simulink model "Accelerator"  (R2022b)
settings: Solver=FixedStepDiscrete  StartTime=0.0  StopTime=10  FixedStep=0.005  RelTol=1e-3  EnableMultiTasking=on
PreLoadFcn:
  | try, model_open; catch, disp('Error occurred while executing model pre-load callback: model_open.m'); disp('Please assure that the MATLAB working directory is set to the model directory before opening.'); end
InitFcn:
  | try, model_open; catch, end
undefined symbols (not defined in the file): GCM, raptor_get_safe_string, raptor_xcp_function
libraries: Raptor_lib x134, simulink x14, Blocks_Library x2, simulink_extras x1
(part 3 of 3)

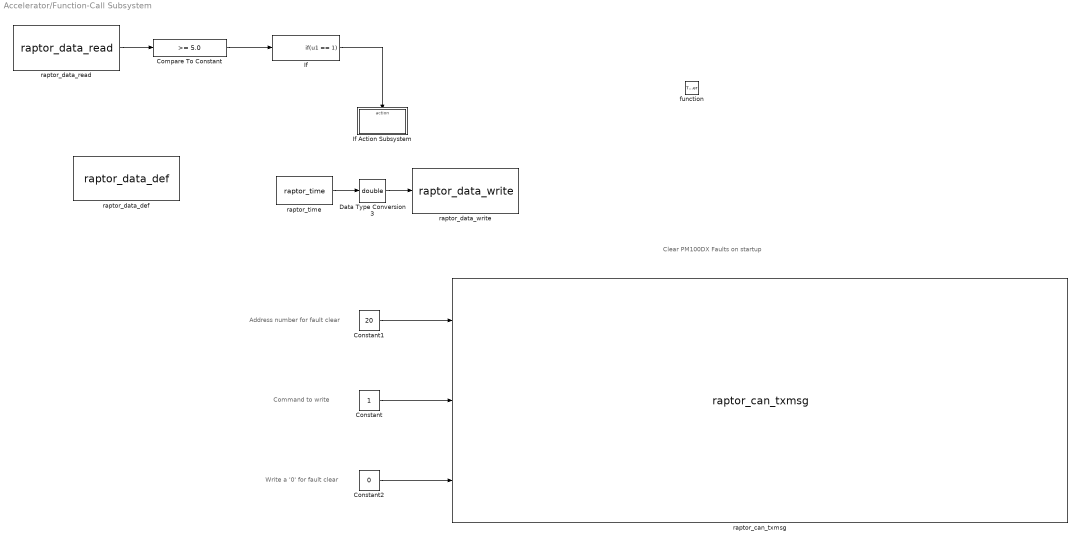
== system Accelerator/Function-Call Subsystem ==
  note: Write a '0' for fault clear
  note: Command to write
  note: Address number for fault clear
  note: Clear PM100DX Faults on startup
  function : TriggerPort  TriggerType=function-call  VariantControl=(inherit)
  Compare To Constant : simulink/Logic and Bit Operations/Compare To Constant  relop=>=  const=5.0  OutDataTypeStr=boolean
  Constant : Constant
  Constant1 : Constant  Value=20
  Constant2 : Constant  Value=0
  Data Type Conversion3 : DataTypeConversion  OutDataTypeStr=double  SaturateOnIntegerOverflow=off  RndMeth=Floor
  If : If  IfExpression=u1 == 1  ShowElse=off
  If Action Subsystem : Subsystem  TreatAsAtomicUnit=on
  raptor_can_txmsg : Raptor_lib/CAN/raptor_can_txmsg  canDefinition=struct('dbcFile', '20210505 RMS PM and RM CAN DB.dbc','message', 'M193_Read_Write_Param_Command','comment', 'Parameter Message sent as needed by VCU to request info, change EEPROM, or command a function.','signals', {{'D1_Parameter_Address_Command','D2_Read_Write_Command','D3_Data_Command'}},'enabled', [ 1 1 1;],'scaled', [ 1 1 1;],'canBus', '''CAN1''','messageID', [ 193;],'idMask', [ 536870911;],'payloadMask', [],'payloadValue', [],'period', [ 0;],'queueSize', [ 1;],'label', [ 0;],'ver', [ 2;],'showID', [ 0;],'showRaw', [ 0;],'showRawMsg', [ 0;],'useStartVals', [ 0;],'useSimFunc', [ 0;],'sim_func_name', '''''','fill', [ 0;],'editID', [ 0;],'signalOrder', [ 1;],'signalAscDes', [ 1;],'msgLength', [ 8;])  canBus='CAN1'  queueSize=1  payloadMask=[]  payloadValue=[]  period=0  showID=0  label=0  idMask=hex2dec('1FFFFFFF')  fill=0  id=193  showRaw=0  signalOrder=1  signalInfo={{struct('Name', 'D3_Data_Command','Startbit', [ 0;],'SignalSize', [ 16;],'ByteOrder', 'LittleEndian','ValueType', 'SIGNED','Class', 'int16','Signed', [ 1;],'Factor', [ 1;],'Offset', [ 0;],'Min', [ -32768;],'Max', [ 32767;],'Units', '','StartVal', [ NaN;],'Comment', 'All EEPROM data is 16 bits and is contained in bytes 4 and 5.','Multiplexed', [ 0;],'Multiplexor', [ 0;],'MultiplexMode_Min', [ 0;],'MultiplexMode_Max', [ 0;],'StartBit', [ 32;]),struct('Name', 'D2_Read_Write_Command','Startbit', [ 0;],'SignalSize', [ 1;],'ByteOrder', 'LittleEndian','ValueType', 'UNSIGNED','Class', 'uint8','Signed', [ 0;],'Factor', [ 1;],'Offset', [ 0;],'Min', [ 0;],'Max', [ 1;],'Units', '','StartVal', [ NaN;],'Comment', '0=Read, 1=Write','Multiplexed', [ 0;],'Multiplexor', [ 0;],'MultiplexMode_Min', [ 0;],'MultiplexMode_Max', [ 0;],'StartBit', [ 16;]),struct('Name', 'D1_Parameter_Address_Command','Startbit', [ 0;],'SignalSize', [ 16;],'ByteOrder', 'LittleEndian','ValueType', 'UNSIGNED','Class', 'uint16','Signed', [ 0;],'Factor', [ 1;],'Offset', [ 0;],'Min', [ 0;],'Max', [ 65535;],'Units', '','StartVal', [ NaN;],'Comment', 'Valid EEPROM Parameter CAN addresses are between 100 and 499.','Multiplexed', [ 0;],'Multiplexor', [ 0;],'MultiplexMode_Min', [ 0;],'MultiplexMode_Max', [ 0;],'StartBit', [ 0;])}}  useSimFunc=0  sim_func_name=''  useStartVals=0
      settings: SourceProductName=Raptor
  raptor_data_def : Raptor_lib/Data Storage/raptor_data_def  dataName='AbsoluteTime'  initValue=0  dataType=double  storage=Volatile (RAM)  calVisible=on  calType=Measurement  calDispType=Number  calEnum={'False', 'True'}  calGain=1.0  calOffset=0  calMin=-inf  calMax=inf  calFormat='-1'  calUnit=''  calHelp=''  calAccess=1  calFunction=raptor_xcp_function(gcb)  calDispHeaders=off  calColHeaders={'Col1' 'Col2' 'Col3'}  calRowHeaders={'Row1' 'Row2' 'Row3'}
      settings: SourceProductName=Raptor
  raptor_data_read : Raptor_lib/Data Storage/raptor_data_read  dataName='AbsoluteTime'  dataShape=Scalar  idxSource=Input  idxRow=1  idxCol=1
      settings: SourceProductName=Raptor
  raptor_data_write : Raptor_lib/Data Storage/raptor_data_write  dataName='AbsoluteTime'  dataShape=Scalar  idxSource=Input Port  idxRow=1  idxCol=1
      settings: SourceProductName=Raptor
  raptor_time : Raptor_lib/Triggers/raptor_time  unit=milliseconds
      settings: SourceProductName=Raptor
  wires:
  raptor_time/1 -> Data Type Conversion3/1
  raptor_data_read/1 -> Compare To Constant/1
  Compare To Constant/1 -> If/1
  If/1 -> If Action Subsystem/Action
  Data Type Conversion3/1 -> raptor_data_write/1
  Constant/1 -> raptor_can_txmsg/2
  Constant1/1 -> raptor_can_txmsg/1
  Constant2/1 -> raptor_can_txmsg/3

== system Accelerator/Power Up_Down ==
  Background : Subsystem
  raptor_timed_trigger : Raptor_lib/Triggers/raptor_timed_trigger  triggerValues=Foreground|Foregroundx2|Foregroundx5|Foregroundx10|Foregroundx20|Background|Backgroundx2|Backgroundx5|Backgroundx10|Backgroundx20|Second|Minute  trigger=Background  inherited=0  alwaysEnabled=1  triggerPriority=50  triggerName=BGND_G6Wyo
      settings: SourceProductName=Raptor
  wires:
  raptor_timed_trigger/1 -> Background/Trigger

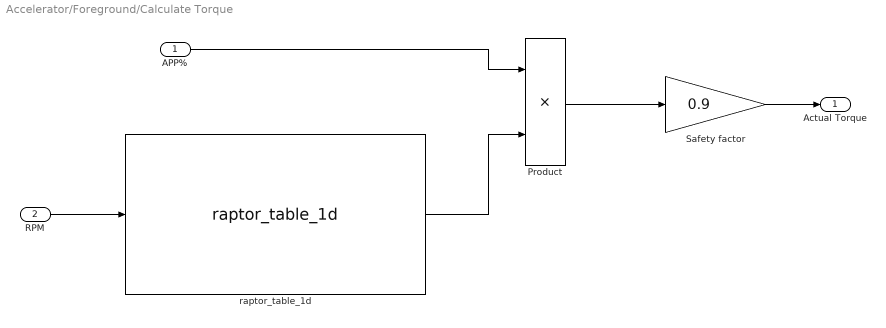
== system Accelerator/Foreground/Calculate Torque ==
  APP% : Inport
  RPM : Inport  Port=2
  Product : Product
  Safety factor : Gain  Gain=0.9
  raptor_table_1d : Raptor_lib/Table Lookup/raptor_table_1d  dataName='MaxTorqueMap'  initValue=|  dataType=double  storage=Calibration  initValueX=|  dataTypeXY=double  storageXY=Calibration  calVisible=on  showTable=on  calGain=1.0  calOffset=0.0  calMax=Inf  calMin=-Inf  calFormat='-1'  calUnit='Nm'  calHelp=''  showBreakpoint=on  dataNameX='RPM'  calGainX=1.0  calOffsetX=0.0  calMaxX=Inf  calMinX=-Inf  calFormatX='-1'  calUnitX='RPM'  calHelpX=''  calAccess=1  calFunction=raptor_xcp_function(gcb)  measureEnable=off  mName=['Data1D_Output']
      initValue=|
      | [72.93410474
      | 73.78666066
      | 74.63821474
      | 75.27137025
      | 76.76910361
      | 77.18486237
      | 78.03541463
      | 78.66957197
      | 79.30372931
      | 79.93588299
      | 80.3466326
      | 80.54499462
      | 80.96075337
      | 80.94171864
      | 80.92368573
      | 80.90465099
      | 80.44481178
      | 80.20838029
      | 79.97194881
      | 79.5191224
      | 78.63050066
      | 77.73586796
      | 77.27602875
      | 75.94660255
      | 75.05798081
      | 74.17036091
      | 73.28173917
      | 72.39411927
      | 70.84729632
      | 69.74127783
      | 68.85365793
      | 67.52423172
      | 66.20081649]
      initValueX=|
      | [1.527788213
      | 158.0133744
      | 323.7157813
      | 498.6851003
      | 719.5381571
      | 894.5575676
      | 1069.476795
      | 1235.229293
      | 1400.981792
      | 1585.167931
      | 1806.271445
      | 1981.340947
      | 2156.360358
      | 2331.479951
      | 2497.382723
      | 2672.502317
      | 2903.023017
      | 3078.192702
      | 3253.362386
      | 3419.365342
      | 3594.685301
      | 3825.306184
      | 4055.826884
      | 4286.54795
      | 4461.867909
      | 4627.971047
      | 4803.291006
      | 4969.394144
      | 5200.165302
      | 5375.535352
      | 5541.63849
      | 5772.359556
      | 5947.779698]
      settings: SourceProductName=Raptor
  Actual Torque : Outport
  wires:
  RPM/1 -> raptor_table_1d/1
  raptor_table_1d/1 -> Product/2
  APP%/1 -> Product/1
  Product/1 -> Safety factor/1
  Safety factor/1 -> Actual Torque/1

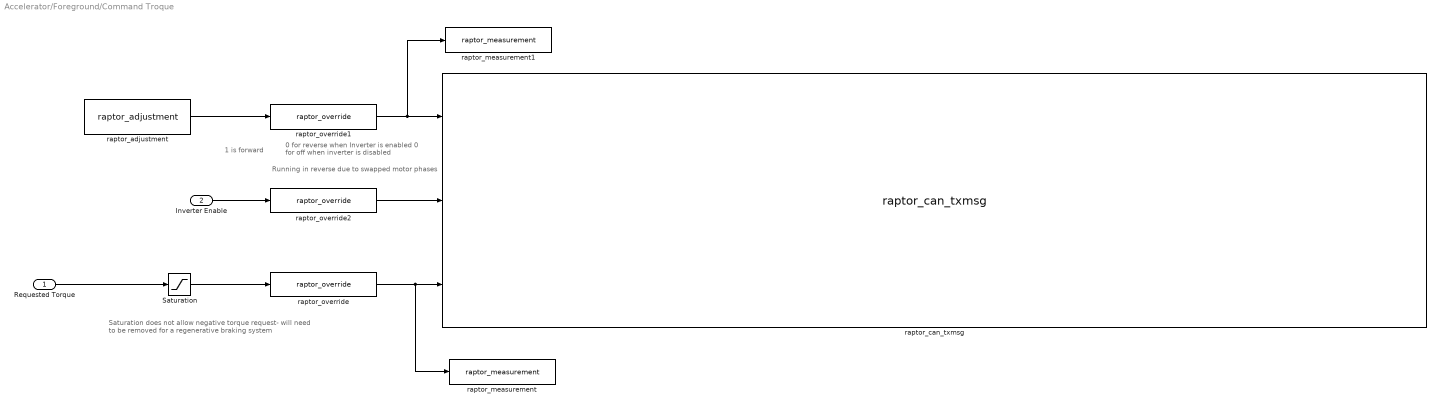
== system Accelerator/Foreground/Command Troque ==
  note: 0 for reverse when Inverter is enabled
      | 0 for off when inverter is disabled
  note: 1 is forward
  note: Saturation does not allow negative torque request-
      | will need to be removed for a regenerative braking system
  note: Running in reverse due to swapped motor phases
  Requested Torque : Inport
  Inverter Enable : Inport  Port=2
  Saturation : Saturate  UpperLimit=3276  LowerLimit=0
  raptor_adjustment : Raptor_lib/Data Storage/raptor_adjustment  paramName='Vehicle_direction'  nameSource=Parameter  initValue=0.00  dataType=double  storage=Calibration  calDispType=Number  calEnum={'False', 'True'}  calGain=1.0  calOffset=0.0  calMax=inf  calMin=-inf  calFormat='-1'  calUnit=''  calHelp=''  calAccess=1  calFunction=raptor_xcp_function(gcb)  calDispHeaders=off  calColHeaders={'Col1' 'Col2' 'Col3'}  calRowHeaders={'Row1' 'Row2' 'Row3'}
      settings: SourceProductName=Raptor
  raptor_can_txmsg : Raptor_lib/CAN/raptor_can_txmsg  canDefinition=struct('dbcFile', '20210505 RMS PM and RM CAN DB.dbc','message', 'M192_Command_Message','comment', 'The command message is used to transmit data to the controller. This message is sent from a user supplied external controller to the PMxxx controller.','signals', {{'Direction_Command','Inverter_Discharge','Inverter_Enable','RollingCounter','Speed_Command','Speed_Mode_Enable','Torque_Command','Torque_Limit_Command'}},'enabled', [ 1 0 1 0 0 0 1 0;],'scaled', [ 1 1 1 1 1 1 1 1;],'canBus', '''CAN1''','messageID', [ 192;],'idMask', [ 536870911;],'payloadMask', [],'payloadValue', [],'period', [ 10;],'queueSize', [ 1;],'label', [ 0;],'ver', [ 2;],'showID', [ 0;],'showRaw', [ 0;],'showRawMsg', [ 0;],'useStartVals', [ 0;],'useSimFunc', [ 0;],'sim_func_name', '''''','fill', [ 0;],'editID', [ 0;],'signalOrder', [ 1;],'signalAscDes', [ 1;],'msgLength', [ 8;])  canBus='CAN1'  queueSize=1  payloadMask=[]  payloadValue=[]  period=10  showID=0  label=0  idMask=hex2dec('1FFFFFFF')  fill=0  id=192  showRaw=0  signalOrder=1  signalInfo={{struct('Name', 'Inverter_Enable','Startbit', [ 0;],'SignalSize', [ 1;],'ByteOrder', 'LittleEndian','ValueType', 'UNSIGNED','Class', 'uint8','Signed', [ 0;],'Factor', [ 1;],'Offset', [ 0;],'Min', [ 0;],'Max', [ 1;],'Units', 'Bit','StartVal', [ NaN;],'Comment', '0=Inverter OFF, 1 = Inverter ON','Multiplexed', [ 0;],'Multiplexor', [ 0;],'MultiplexMode_Min', [ 0;],'MultiplexMode_Max', [ 0;],'StartBit', [ 40;]),struct('Name', 'Direction_Command','Startbit', [ 0;],'SignalSize', [ 1;],'ByteOrder', 'LittleEndian','ValueType', 'UNSIGNED','Class', 'uint8','Signed', [ 0;],'Factor', [ 1;],'Offset', [ 0;],'Min', [ 0;],'Max', [ 1;],'Units', 'Bit','StartVal', [ NaN;],'Comment', '0=CW, 1=CCW as veiwed from the shaft end of the motor','Multiplexed', [ 0;],'Multiplexor', [ 0;],'MultiplexMode_Min', [ 0;],'MultiplexMode_Max', [ 0;],'StartBit', [ 32;]),struct('Name', 'Speed_Command','Startbit', [ 0;],'SignalSize', [ 16;],'ByteOrder', 'LittleEndian','ValueType', 'SIGNED','Class', 'int16','Signed', [ 1;],'Factor', [ 1;],'Offset', [ 0;],'Min', [ -32768;],'Max', [ 32767;],'Units', 'rpm','StartVal', [ NaN;],'Comment', 'Speed commandused when in speed mode','Multiplexed', [ 0;],'Multiplexor', [ 0;],'MultiplexMode_Min', [ 0;],'MultiplexMode_Max', [ 0;],'StartBit', [ 16;]),struct('Name', 'Torque_Command','Startbit', [ 0;],'SignalSize', [ 16;],'ByteOrder', 'LittleEndian','ValueType', 'SIGNED','Class', 'int16','Signed', [ 1;],'Factor', [ 0.1;],'Offset', [ 0;],'Min', [ -3276.8;],'Max', [ 3276.7;],'Units', 'Nm','StartVal', [ NaN;],'Comment', 'Torque command when in torque mode','Multiplexed', [ 0;],'Multiplexor', [ 0;],'MultiplexMode_Min', [ 0;],'MultiplexMode_Max', [ 0;],'StartBit', [ 0;]),struct('Name', 'Inverter_Discharge','Startbit', [ 0;],'SignalSize', [ 1;],'ByteOrder', 'LittleEndian','ValueType', 'UNSIGNED','Class', 'uint8','Signed', [ 0;],'Factor', [ 1;],'Offset', [ 0;],'Min', [ 0;],'Max', [ 1;],'Units', 'Bit','StartVal', [ NaN;],'Comment', '0=Discharge Disable,','Multiplexed', [ 0;],'Multiplexor', [ 0;],'MultiplexMode_Min', [ 0;],'MultiplexMode_Max', [ 0;],'StartBit', [ 41;]),struct('Name', 'Torque_Limit_Command','Startbit', [ 0;],'SignalSize', [ 16;],'ByteOrder', 'LittleEndian','ValueType', 'SIGNED','Class', 'int16','Signed', [ 1;],'Factor', [ 0.1;],'Offset', [ 0;],'Min', [ -3276.8;],'Max', [ 3276.7;],'Units', 'Nm','StartVal', [ NaN;],'Comment', 'Torque Limit, set to 0 to keep default','Multiplexed', [ 0;],'Multiplexor', [ 0;],'MultiplexMode_Min', [ 0;],'MultiplexMode_Max', [ 0;],'StartBit', [ 48;]),struct('Name', 'Speed_Mode_Enable','Startbit', [ 0;],'SignalSize', [ 1;],'ByteOrder', 'LittleEndian','ValueType', 'UNSIGNED','Class', 'uint8','Signed', [ 0;],'Factor', [ 1;],'Offset', [ 0;],'Min', [ 0;],'Max', [ 1;],'Units', 'Bit','StartVal', [ NaN;],'Comment', '0 = No change to mode, 1 = change to speed mode from torque mode','Multiplexed', [ 0;],'Multiplexor', [ 0;],'MultiplexMode_Min', [ 0;],'MultiplexMode_Max', [ 0;],'StartBit', [ 42;]),struct('Name', 'RollingCounter','Startbit', [ 0;],'SignalSize', [ 4;],'ByteOrder', 'LittleEndian','ValueType', 'UNSIGNED','Class', 'uint8','Signed', [ 0;],'Factor', [ 1;],'Offset', [ 0;],'Min', [ 0;],'Max', [ 15;],'Units', 'Bits','StartVal', [ NaN;],'Comment', 'Rolling Counter command','Multiplexed', [ 0;],'Multiplexor', [ 0;],'MultiplexMode_Min', [ 0;],'MultiplexMode_Max', [ 0;],'StartBit', [ 44;])}}  useSimFunc=0  sim_func_name=''  useStartVals=0
      settings: SourceProductName=Raptor
  raptor_measurement : Raptor_lib/Data Storage/raptor_measurement  paramName='Torque_cmd'  nameSource=Parameter  calDispType=Number  calEnum={'False', 'True'}  calGain=1.0  calOffset=0.0  calMax=inf  calMin=-inf  calFormat='-1'  calUnit=''  calHelp=''  calAccess=1  calFunction=raptor_xcp_function(gcb)  calVisible=on
      settings: SourceProductName=Raptor
  raptor_measurement1 : Raptor_lib/Data Storage/raptor_measurement  paramName='Direction_cmd'  nameSource=Parameter  calDispType=Number  calEnum={'False', 'True'}  calGain=1.0  calOffset=0.0  calMax=inf  calMin=-inf  calFormat='-1'  calUnit=''  calHelp=''  calAccess=1  calFunction=raptor_xcp_function(gcb)  calVisible=on
      settings: SourceProductName=Raptor
  raptor_override : Raptor_lib/Data Storage/raptor_override  paramName='Torque_cmd_override'  nameSource=Parameter  measurement=None  calDispType=Number  calEnum={'False', 'True'}  calGain=1.0  calOffset=0.0  calMax=inf  calMin=-inf  calFormat='-1'  calUnit=''  calHelp=''  calAccess=1  calFunction="[raptor_xcp_function(gcb) '|'  'Override']"
      settings: SourceProductName=Raptor
  raptor_override1 : Raptor_lib/Data Storage/raptor_override  paramName='Direction_cmd_override'  nameSource=Parameter  measurement=None  calDispType=Number  calEnum={'False', 'True'}  calGain=1.0  calOffset=0.0  calMax=inf  calMin=-inf  calFormat='-1'  calUnit=''  calHelp=''  calAccess=1  calFunction="[raptor_xcp_function(gcb) '|'  'Override']"
      settings: SourceProductName=Raptor
  raptor_override2 : Raptor_lib/Data Storage/raptor_override  paramName='Inverter_enb_override'  nameSource=Parameter  measurement=None  calDispType=Number  calEnum={'False', 'True'}  calGain=1.0  calOffset=0.0  calMax=inf  calMin=-inf  calFormat='-1'  calUnit=''  calHelp=''  calAccess=1  calFunction="[raptor_xcp_function(gcb) '|'  'Override']"
      settings: SourceProductName=Raptor
  wires:
  raptor_adjustment/1 -> raptor_override1/1
  Inverter Enable/1 -> raptor_override2/1
  Requested Torque/1 -> Saturation/1
  raptor_override/1 -> raptor_can_txmsg/3, raptor_measurement/1
  Saturation/1 -> raptor_override/1
  raptor_override1/1 -> raptor_can_txmsg/1, raptor_measurement1/1
  raptor_override2/1 -> raptor_can_txmsg/2

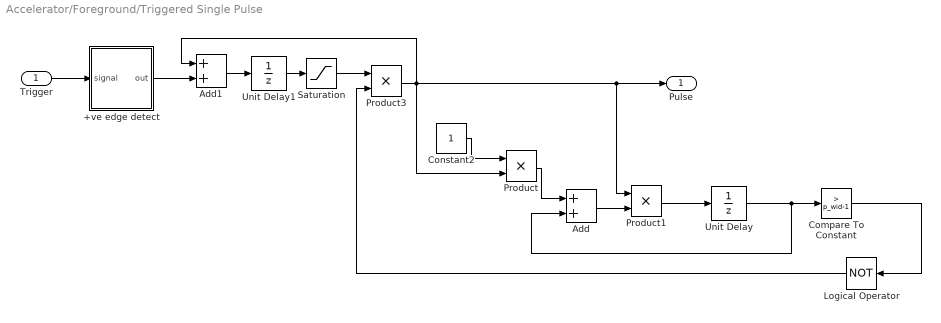
== system Accelerator/Foreground/Triggered Single Pulse ==
  Trigger : Inport
  +ve edge detect : Subsystem
  Add : Sum
  Add1 : Sum
  Compare To Constant : simulink/Logic and Bit Operations/Compare To Constant  relop=>  const=p_wid-1  OutDataTypeStr=boolean
  Constant2 : Constant
  Logical Operator : Logic  Operator=NOT  AllPortsSameDT=off  OutDataTypeStr=boolean
  Product : Product  RndMeth=Zero
  Product1 : Product  RndMeth=Zero
  Product3 : Product  RndMeth=Zero
  Saturation : Saturate  UpperLimit=1  LowerLimit=0
  Unit Delay : UnitDelay  SampleTime=-1  HasFrameUpgradeWarning=on
  Unit Delay1 : UnitDelay  SampleTime=-1  HasFrameUpgradeWarning=on
  Pulse : Outport
  wires:
  Compare To Constant/1 -> Logical Operator/1
  Constant2/1 -> Product/1
  Product/1 -> Add/1
  Unit Delay/1 -> Add/2, Compare To Constant/1
  Trigger/1 -> +ve edge detect/1(signal)
  +ve edge detect/1(out) -> Add1/2
  Add/1 -> Product1/2
  Product1/1 -> Unit Delay/1
  Add1/1 -> Unit Delay1/1
  Unit Delay1/1 -> Saturation/1
  Saturation/1 -> Product3/1
  Product3/1 -> Add1/1, Product/2, Product1/1, Pulse/1
  Logical Operator/1 -> Product3/2

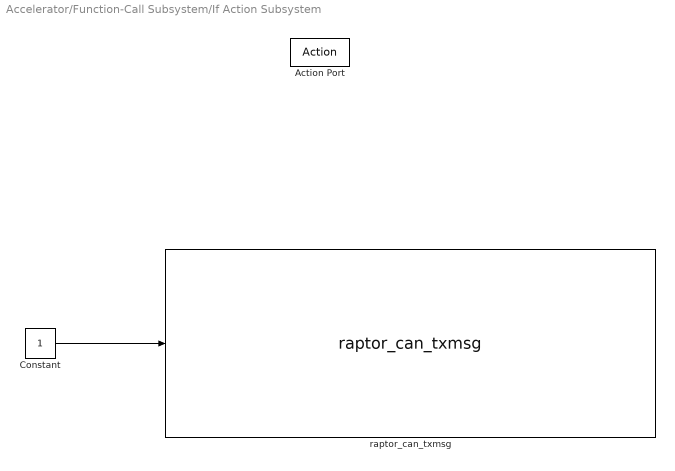
== system Accelerator/Function-Call Subsystem/If Action Subsystem ==
  Action Port : ActionPort  ActionPortLabel=if(u1 == 1)
  Constant : Constant
  raptor_can_txmsg : Raptor_lib/CAN/raptor_can_txmsg  canDefinition=struct('dbcFile', '20210505 RMS PM and RM CAN DB.dbc','message', 'M192_Command_Message','comment', 'The command message is used to transmit data to the controller. This message is sent from a user supplied external controller to the PMxxx controller.','signals', {{'Direction_Command','Inverter_Discharge','Inverter_Enable','RollingCounter','Speed_Command','Speed_Mode_Enable','Torque_Command','Torque_Limit_Command'}},'enabled', [ 0 0 1 0 0 0 0 0;],'scaled', [ 1 1 1 1 1 1 1 1;],'canBus', '''CAN1''','messageID', [ 192;],'idMask', [ 536870911;],'payloadMask', [],'payloadValue', [],'period', [ 0;],'queueSize', [ 1;],'label', [ 0;],'ver', [ 2;],'showID', [ 0;],'showRaw', [ 0;],'showRawMsg', [ 0;],'useStartVals', [ 0;],'useSimFunc', [ 0;],'sim_func_name', '''''','fill', [ 0;],'editID', [ 0;],'signalOrder', [ 1;],'signalAscDes', [ 1;],'msgLength', [ 8;])  canBus='CAN1'  queueSize=1  payloadMask=[]  payloadValue=[]  period=0  showID=0  label=0  idMask=hex2dec('1FFFFFFF')  fill=0  id=192  showRaw=0  signalOrder=1  signalInfo={{struct('Name', 'Inverter_Enable','Startbit', [ 0;],'SignalSize', [ 1;],'ByteOrder', 'LittleEndian','ValueType', 'UNSIGNED','Class', 'uint8','Signed', [ 0;],'Factor', [ 1;],'Offset', [ 0;],'Min', [ 0;],'Max', [ 1;],'Units', 'Bit','StartVal', [ NaN;],'Comment', '0=Inverter OFF, 1 = Inverter ON','Multiplexed', [ 0;],'Multiplexor', [ 0;],'MultiplexMode_Min', [ 0;],'MultiplexMode_Max', [ 0;],'StartBit', [ 40;]),struct('Name', 'Direction_Command','Startbit', [ 0;],'SignalSize', [ 1;],'ByteOrder', 'LittleEndian','ValueType', 'UNSIGNED','Class', 'uint8','Signed', [ 0;],'Factor', [ 1;],'Offset', [ 0;],'Min', [ 0;],'Max', [ 1;],'Units', 'Bit','StartVal', [ NaN;],'Comment', '0=CW, 1=CCW as veiwed from the shaft end of the motor','Multiplexed', [ 0;],'Multiplexor', [ 0;],'MultiplexMode_Min', [ 0;],'MultiplexMode_Max', [ 0;],'StartBit', [ 32;]),struct('Name', 'Speed_Command','Startbit', [ 0;],'SignalSize', [ 16;],'ByteOrder', 'LittleEndian','ValueType', 'SIGNED','Class', 'int16','Signed', [ 1;],'Factor', [ 1;],'Offset', [ 0;],'Min', [ -32768;],'Max', [ 32767;],'Units', 'rpm','StartVal', [ NaN;],'Comment', 'Speed commandused when in speed mode','Multiplexed', [ 0;],'Multiplexor', [ 0;],'MultiplexMode_Min', [ 0;],'MultiplexMode_Max', [ 0;],'StartBit', [ 16;]),struct('Name', 'Torque_Command','Startbit', [ 0;],'SignalSize', [ 16;],'ByteOrder', 'LittleEndian','ValueType', 'SIGNED','Class', 'int16','Signed', [ 1;],'Factor', [ 0.1;],'Offset', [ 0;],'Min', [ -3276.8;],'Max', [ 3276.7;],'Units', 'Nm','StartVal', [ NaN;],'Comment', 'Torque command when in torque mode','Multiplexed', [ 0;],'Multiplexor', [ 0;],'MultiplexMode_Min', [ 0;],'MultiplexMode_Max', [ 0;],'StartBit', [ 0;]),struct('Name', 'Inverter_Discharge','Startbit', [ 0;],'SignalSize', [ 1;],'ByteOrder', 'LittleEndian','ValueType', 'UNSIGNED','Class', 'uint8','Signed', [ 0;],'Factor', [ 1;],'Offset', [ 0;],'Min', [ 0;],'Max', [ 1;],'Units', 'Bit','StartVal', [ NaN;],'Comment', '0=Discharge Disable,','Multiplexed', [ 0;],'Multiplexor', [ 0;],'MultiplexMode_Min', [ 0;],'MultiplexMode_Max', [ 0;],'StartBit', [ 41;]),struct('Name', 'Torque_Limit_Command','Startbit', [ 0;],'SignalSize', [ 16;],'ByteOrder', 'LittleEndian','ValueType', 'SIGNED','Class', 'int16','Signed', [ 1;],'Factor', [ 0.1;],'Offset', [ 0;],'Min', [ -3276.8;],'Max', [ 3276.7;],'Units', 'Nm','StartVal', [ NaN;],'Comment', 'Torque Limit, set to 0 to keep default','Multiplexed', [ 0;],'Multiplexor', [ 0;],'MultiplexMode_Min', [ 0;],'MultiplexMode_Max', [ 0;],'StartBit', [ 48;]),struct('Name', 'Speed_Mode_Enable','Startbit', [ 0;],'SignalSize', [ 1;],'ByteOrder', 'LittleEndian','ValueType', 'UNSIGNED','Class', 'uint8','Signed', [ 0;],'Factor', [ 1;],'Offset', [ 0;],'Min', [ 0;],'Max', [ 1;],'Units', 'Bit','StartVal', [ NaN;],'Comment', '0 = No change to mode, 1 = change to speed mode from torque mode','Multiplexed', [ 0;],'Multiplexor', [ 0;],'MultiplexMode_Min', [ 0;],'MultiplexMode_Max', [ 0;],'StartBit', [ 42;]),struct('Name', 'RollingCounter','Startbit', [ 0;],'SignalSize', [ 4;],'ByteOrder', 'LittleEndian','ValueType', 'UNSIGNED','Class', 'uint8','Signed', [ 0;],'Factor', [ 1;],'Offset', [ 0;],'Min', [ 0;],'Max', [ 15;],'Units', 'Bits','StartVal', [ NaN;],'Comment', 'Rolling Counter command','Multiplexed', [ 0;],'Multiplexor', [ 0;],'MultiplexMode_Min', [ 0;],'MultiplexMode_Max', [ 0;],'StartBit', [ 44;])}}  useSimFunc=0  sim_func_name=''  useStartVals=0
      settings: SourceProductName=Raptor
  wires:
  Constant/1 -> raptor_can_txmsg/1

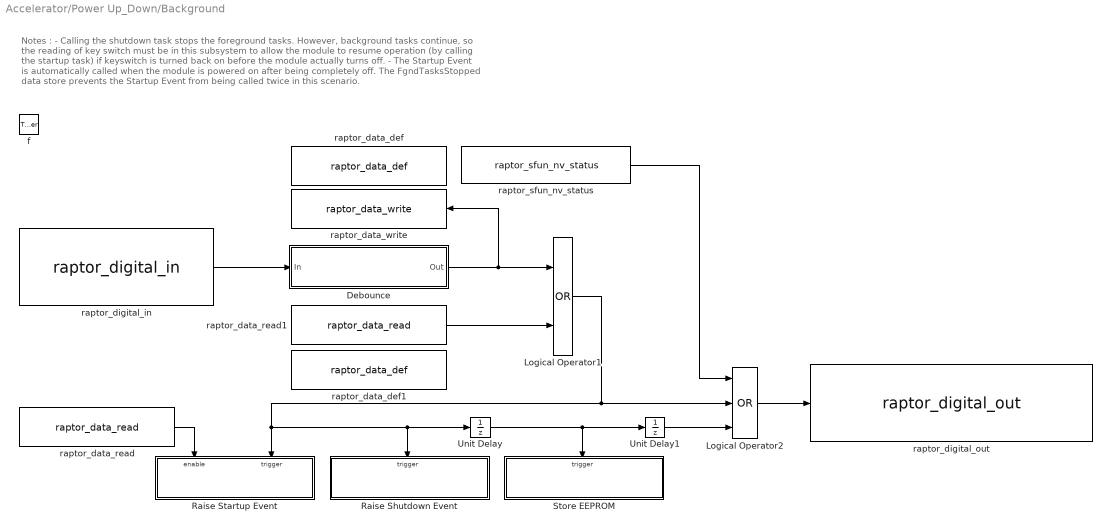
== system Accelerator/Power Up_Down/Background ==
  note: Notes :
      | - Calling the shutdown task stops the foreground tasks. However, background tasks continue, so the reading of key switch must be in this subsystem to allow the module
      | to resume operation (by calling the startup task) if keyswitch is turned back on before the module actually turns off.
      | - The Startup Event is automatically called when the module is powered on after being completely off. The FgndTasksStopped data store prevents the Startup Event from being called twice in this scenario.
  f : TriggerPort  TriggerType=function-call  VariantControl=Variant  ZeroCross=off
  Debounce : Subsystem
  Logical Operator1 : Logic  Operator=OR  OutDataTypeStr=boolean
  Logical Operator2 : Logic  Operator=OR  Inputs=3  OutDataTypeStr=boolean
  Raise Shutdown Event : Subsystem  TreatAsAtomicUnit=on
  Raise Startup Event : Subsystem  TreatAsAtomicUnit=on
  Store EEPROM : Subsystem  TreatAsAtomicUnit=on
  Unit Delay : UnitDelay  SampleTime=-1  HasFrameUpgradeWarning=on
  Unit Delay1 : UnitDelay  SampleTime=-1  HasFrameUpgradeWarning=on
  raptor_data_def : Raptor_lib/Data Storage/raptor_data_def  dataName='KeySw_Bgnd'  initValue=0  dataType=boolean  storage=Volatile (RAM)  calVisible=on  calType=Measurement  calDispType=Number  calEnum={'False', 'True'}  calGain=1.0  calOffset=0  calMin=-Inf  calMax=Inf  calFormat='-1'  calUnit='Bool'  calHelp='Key switch reading from background task'  calAccess=1  calFunction=group  calDispHeaders=off  calColHeaders={'Col1' 'Col2' 'Col3'}  calRowHeaders={'Row1' 'Row2' 'Row3'}
      settings: SourceProductName=Raptor
  raptor_data_def1 : Raptor_lib/Data Storage/raptor_data_def  dataName='KeepModuleOn'  initValue=0  dataType=boolean  storage=Volatile (RAM)  calVisible=on  calType=Measurement  calDispType=Number  calEnum={'False', 'True'}  calGain=1.0  calOffset=0  calMin=-Inf  calMax=Inf  calFormat='-1'  calUnit='Bool'  calHelp='Boolean indicating module to be kept on'  calAccess=1  calFunction=group  calDispHeaders=off  calColHeaders={'Col1' 'Col2' 'Col3'}  calRowHeaders={'Row1' 'Row2' 'Row3'}
      settings: SourceProductName=Raptor
  raptor_data_read : Raptor_lib/Data Storage/raptor_data_read  dataName='FgndTasksStopped'  dataShape=Scalar  idxSource=Input  idxRow=1  idxCol=1
      settings: SourceProductName=Raptor
  raptor_data_read1 : Raptor_lib/Data Storage/raptor_data_read  dataName='KeepModuleOn'  dataShape=Scalar  idxSource=Input  idxRow=1  idxCol=1
      settings: SourceProductName=Raptor
  raptor_data_write : Raptor_lib/Data Storage/raptor_data_write  dataName='KeySw_Bgnd'  dataShape=Scalar  idxSource=Input Port  idxRow=1  idxCol=1
      settings: SourceProductName=Raptor
  raptor_digital_in : Raptor_lib/Input & Output/raptor_digital_in  resourceValues=(None)|WAKE_INPUT1|INPUT33|INPUT34|INPUT35|INPUT36|INPUT37|INPUT38|INPUT39|INPUT40  resource=WAKE_INPUT1  pullUDValues=2.9k PD  pullUD=2.9k PD  upperThres=1.980  lowerThres=1.320
      settings: SourceProductName=Raptor
  raptor_digital_out : Raptor_lib/Input & Output/raptor_digital_out  resourceValues=OUTPUT9|OUTPUT21|OUTPUT22|OUTPUT23|OUTPUT24|(None)|OUTPUT1|OUTPUT2|OUTPUT3|OUTPUT4|OUTPUT5|OUTPUT6|OUTPUT7|OUTPUT8|OUTPUT10|OUTPUT11|OUTPUT25|OUTPUT26|OUTPUT27|OUTPUT28|OUTPUT29|OUTPUT30|OUTPUT31|OUTPUT32|OUTPUT33|OUTPUT34|OUTPUT35|OUTPUT36|OUTPUT37|OUTPUT38|OUTPUT39|OUTPUT40|OUTPUT41|OUTPUT42|OUTPUT43|OUTPUT44|OUTPUT45|OUTPUT46|OUTPUT47|OUTPUT48|POWER_HOLD  resource=POWER_HOLD  driverTypeValues=(None)  driverType=(None)
      settings: SourceProductName=Raptor
  raptor_sfun_nv_status : Raptor_lib/Data Storage/raptor_sfun_nv_status  showStatus=Store In Progess
      settings: SourceProductName=Raptor
  wires:
  raptor_data_read/1 -> Raise Startup Event/Enable
  raptor_digital_in/1 -> Debounce/1(In)
  Logical Operator2/1 -> raptor_digital_out/1
  Unit Delay/1 -> Store EEPROM/Trigger, Unit Delay1/1
  Logical Operator1/1 -> Logical Operator2/2, Raise Startup Event/Trigger, Raise Shutdown Event/Trigger, Unit Delay/1
  Unit Delay1/1 -> Logical Operator2/3
  raptor_sfun_nv_status/1 -> Logical Operator2/1
  raptor_data_read1/1 -> Logical Operator1/2
  Debounce/1(Out) -> raptor_data_write/1, Logical Operator1/1

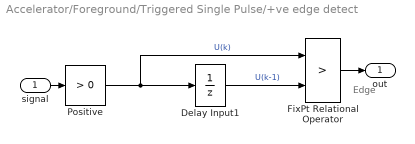
== system Accelerator/Foreground/Triggered Single Pulse/+ve edge detect ==
  note: Edge
  signal : Inport
  Delay Input1 : UnitDelay  Description=Store in Global RAM  DisableCoverage=on  SampleTime=-1  HasFrameUpgradeWarning=on
  FixPt Relational Operator : RelationalOperator  Operator=>  OutDataTypeStr=fixdt(0, 8)  ZeroCross=off  InputSameDT=off
  Positive : simulink/Logic and Bit Operations/Compare To Zero  relop=>  OutDataTypeStr=uint8  ZeroCross=off
  out : Outport
  wires:
  Delay Input1/1 -> FixPt Relational Operator/2  "U(k-1)"
  Positive/1 -> Delay Input1/1, FixPt Relational Operator/1  "U(k)"
  FixPt Relational Operator/1 -> out/1
  signal/1 -> Positive/1

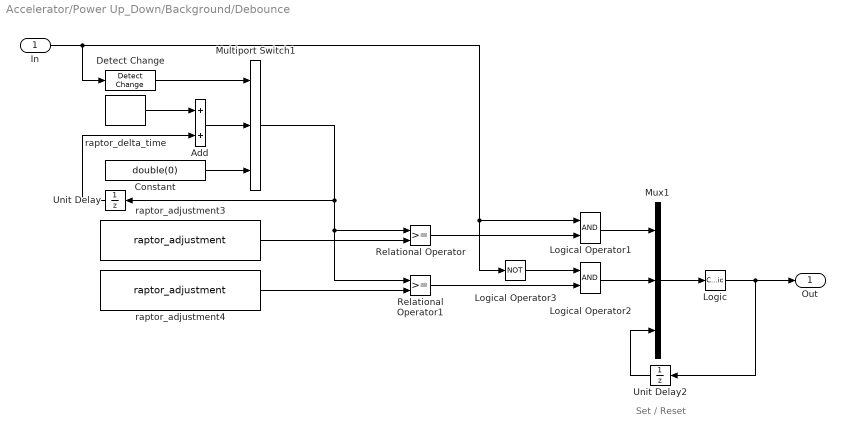
== system Accelerator/Power Up_Down/Background/Debounce ==
  note: Set / Reset
  In : Inport
  Add : Sum
  Constant : Constant  Value=double(0)
  Detect Change : simulink/Logic and Bit Operations/Detect Change  vinit=0  OutDataTypeStr=boolean
  Logic : CombinatorialLogic  TruthTable=[0;1;0;0;1;1;0;0]
  Logical Operator1 : Logic  AllPortsSameDT=off  OutDataTypeStr=boolean
  Logical Operator2 : Logic  AllPortsSameDT=off  OutDataTypeStr=boolean
  Logical Operator3 : Logic  Operator=NOT  Inputs=1  AllPortsSameDT=off  OutDataTypeStr=boolean
  Multiport Switch1 : MultiPortSwitch  DataPortOrder=Zero-based contiguous  Inputs=2  zeroidx=on  SaturateOnIntegerOverflow=off  InputSameDT=off
  Mux1 : Mux  Inputs=3
  Relational Operator : RelationalOperator  OutDataTypeStr=boolean  InputSameDT=off
  Relational Operator1 : RelationalOperator  OutDataTypeStr=boolean  InputSameDT=off
  Unit Delay : UnitDelay  SampleTime=-1  HasFrameUpgradeWarning=on
  Unit Delay2 : UnitDelay  InitialCondition=1  SampleTime=-1  HasFrameUpgradeWarning=on
  raptor_adjustment3 : Raptor_lib/Data Storage/raptor_adjustment  paramName='KeySwHiTimeThr'  nameSource=Parameter  initValue=0.2  dataType=double  storage=Calibration  calDispType=Number  calEnum={'Active Low', 'Active High'}  calGain=1  calOffset=0  calMax=inf  calMin=-inf  calFormat='-1'  calUnit='sec'  calHelp='State high time threshold'  calAccess=1  calFunction=group  calDispHeaders=off  calColHeaders={'Col1' 'Col2' 'Col3'}  calRowHeaders={'Row1' 'Row2' 'Row3'}
      settings: SourceProductName=Raptor
  raptor_adjustment4 : Raptor_lib/Data Storage/raptor_adjustment  paramName='KeySwLoTimeThr'  nameSource=Parameter  initValue=0.2  dataType=double  storage=Calibration  calDispType=Number  calEnum={'Active Low', 'Active High'}  calGain=1  calOffset=0  calMax=inf  calMin=-inf  calFormat='-1'  calUnit='sec'  calHelp='State low time threshold'  calAccess=1  calFunction=group  calDispHeaders=off  calColHeaders={'Col1' 'Col2' 'Col3'}  calRowHeaders={'Row1' 'Row2' 'Row3'}
      settings: SourceProductName=Raptor
  raptor_delta_time : Raptor_lib/Triggers/raptor_delta_time  unit=seconds
      settings: SourceProductName=Raptor
  Out : Outport  VectorParamsAs1DForOutWhenUnconnected=off
  wires:
  Detect Change/1 -> Multiport Switch1/1
  Logical Operator3/1 -> Logical Operator2/1
  Relational Operator/1 -> Logical Operator1/2
  Logical Operator2/1 -> Mux1/2
  Logical Operator1/1 -> Mux1/1
  Mux1/1 -> Logic/1
  Unit Delay2/1 -> Mux1/3
  In/1 -> Detect Change/1, Logical Operator1/1, Logical Operator3/1
  Multiport Switch1/1 -> Unit Delay/1, Relational Operator/1, Relational Operator1/1
  Add/1 -> Multiport Switch1/2
  Constant/1 -> Multiport Switch1/3
  Relational Operator1/1 -> Logical Operator2/2
  Logic/1 -> Unit Delay2/1, Out/1
  Unit Delay/1 -> Add/2
  raptor_delta_time/1 -> Add/1
  raptor_adjustment4/1 -> Relational Operator1/2
  raptor_adjustment3/1 -> Relational Operator/2

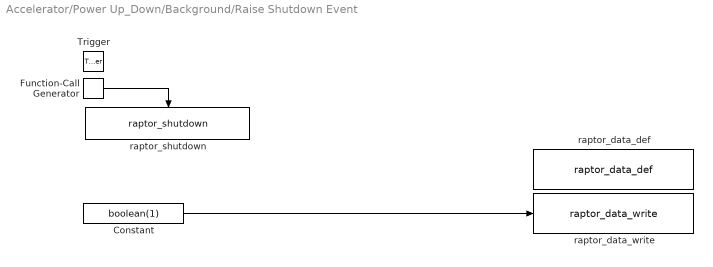
== system Accelerator/Power Up_Down/Background/Raise Shutdown Event ==
  Trigger : TriggerPort  TriggerType=falling  VariantControl=Variant
  Constant : Constant  Value=boolean(1)
  Function-Call Generator : simulink/Ports & Subsystems/Function-Call Generator  sample_time=-1  numberOfIterations=1  DisallowWideOutput=off
  raptor_data_def : Raptor_lib/Data Storage/raptor_data_def  dataName='FgndTasksStopped'  initValue=0  dataType=boolean  storage=Volatile (RAM)  calVisible=on  calType=Measurement  calDispType=Number  calEnum={'False', 'True'}  calGain=1.0  calOffset=0  calMin=-Inf  calMax=Inf  calFormat='-1'  calUnit='Bool'  calHelp='Boolean indicating foreground tasks stopped'  calAccess=1  calFunction=group  calDispHeaders=off  calColHeaders={'Col1' 'Col2' 'Col3'}  calRowHeaders={'Row1' 'Row2' 'Row3'}
      settings: SourceProductName=Raptor
  raptor_data_write : Raptor_lib/Data Storage/raptor_data_write  dataName='FgndTasksStopped'  dataShape=Scalar  idxSource=Input Port  idxRow=1  idxCol=1
      settings: SourceProductName=Raptor
  raptor_shutdown : Raptor_lib/Triggers/raptor_shutdown  null=0
      settings: SourceProductName=Raptor
  wires:
  Constant/1 -> raptor_data_write/1
  Function-Call Generator/1 -> raptor_shutdown/Trigger

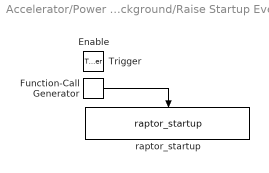
== system Accelerator/Power Up_Down/Background/Raise Startup Event ==
  Enable : EnablePort
  Trigger : TriggerPort  VariantControl=Variant
  Function-Call Generator : simulink/Ports & Subsystems/Function-Call Generator  sample_time=-1  numberOfIterations=1  DisallowWideOutput=off
  raptor_startup : Raptor_lib/Triggers/raptor_startup  null=0
      settings: SourceProductName=Raptor
  wires:
  Function-Call Generator/1 -> raptor_startup/Trigger

== system Accelerator/Power Up_Down/Background/Store EEPROM ==
  Trigger : TriggerPort  TriggerType=falling  VariantControl=Variant
  Function-Call Generator : simulink/Ports & Subsystems/Function-Call Generator  sample_time=-1  numberOfIterations=1  DisallowWideOutput=off
  raptor_store_nv : Raptor_lib/Data Storage/raptor_store_nv  null=0
      settings: SourceProductName=Raptor
  wires:
  Function-Call Generator/1 -> raptor_store_nv/Trigger

== matlab function Accelerator/Foreground/MATLAB Function ==
  data: u input; y output
function y = fcn(u)
y = abs(u(2)-u(1));
end

== matlab function Accelerator/Foreground/MATLAB Function2 ==
  data: u input; y output
function y = fcn(u)
y = u/4095*100;
end

== matlab function Accelerator/Foreground/MATLAB Function1 ==
  data: u input; y output
function y = fcn(u)
y = (u(2)+u(1))/2;
end
